simulink model "model243"  (R2024b)
settings: Solver=VariableStepAuto  StartTime=0.0  StopTime=10.0  RelTol=1e-3
settings Model: Creator=Xist  LastModifiedBy=Xist

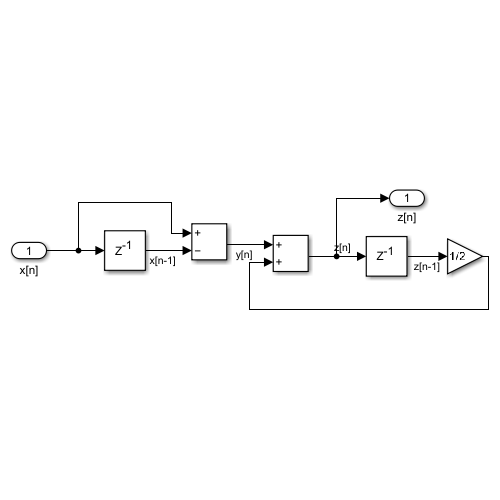
[thumbnail: Simulink's stored preview of the top-level diagram]
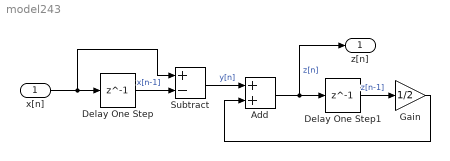
== system model243 ==
  x[n] : Inport
  Add : Sum
  Delay One Step : Delay  DelayLength=1
  Delay One Step1 : Delay  DelayLength=1
  Gain : Gain  Gain=1/2
  Subtract : Sum  Inputs=+-
  z[n] : Outport
  wires:
  x[n]/1 -> Subtract/1, Delay One Step/1
  Subtract/1 -> Add/1  "y[n]"
  Delay One Step/1 -> Subtract/2  "x[n-1]"
  Delay One Step1/1 -> Gain/1  "z[n-1]"
  Add/1 -> Delay One Step1/1, z[n]/1  "z[n]"
  Gain/1 -> Add/2
